simulink model "SIFT_final"  (R2015a)
settings: Solver=ode45  StartTime=0.0  StopTime=10.0  RelTol=1e-3
InitFcn:
  | %% DSPBuilder Start
  | alt_dspbuilder_update_model(bdroot)
  | %% DSPBuilder End
libraries: allblocks_alteradspbuilder2 x1826
(part 1 of 24)
settings Model: Creator=ASUS  LastModifiedBy=ASUS

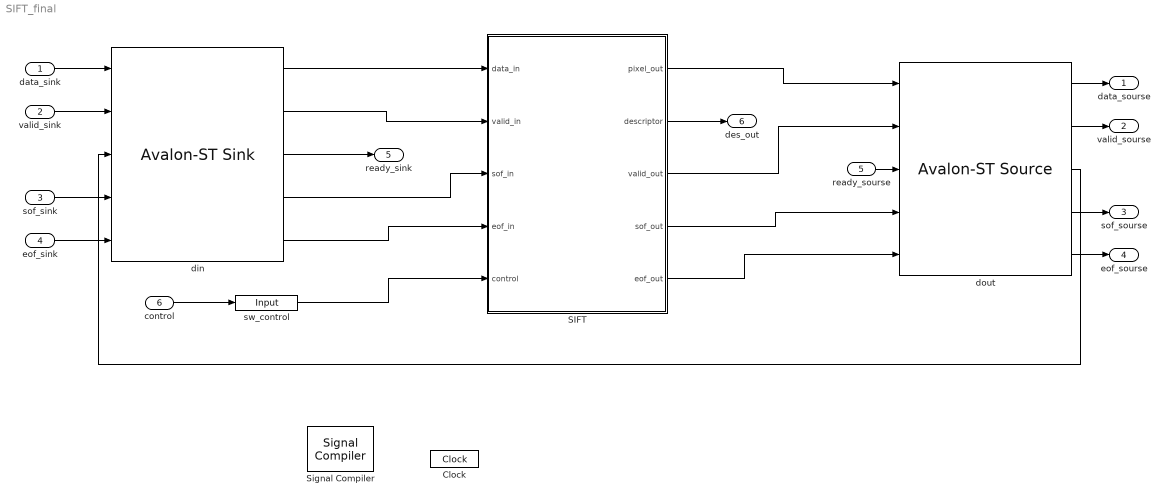
== system SIFT_final ==
  data_sink : Inport
  valid_sink : Inport  Port=2
  sof_sink : Inport  Port=3
  eof_sink : Inport  Port=4
  ready_sourse : Inport  Port=5
  control : Inport  Port=6
  Clock : allblocks_alteradspbuilder2/Clock  ClockPeriod=10/1.5  ClockPeriodUnit=ns  SampleTime=1  ResetLatency=0  ResetRegisterCascadeDepth=0  SimulationStartCycle=5  PhaseOffset=0  Reset=aclr  ResetType=Active Low  Export=off
  SIFT : Subsystem
  Signal Compiler : allblocks_alteradspbuilder2/Signal Compiler  DeviceFamily=Cyclone IV GX  DeviceName=AUTO  DisableEarlyHDLGeneration=off  EnableSignalTap=on  SignalTapDepth=256  UseBoardBlock=off  StpUseDefaultClock=on  StpClock=Clock  ExportDir=C:\altera\16.0\quartus\dsp_builder  MAX10_ProgrammingMode=Internal Flash (SDM) Single Boot
  din : allblocks_alteradspbuilder2/Avalon-ST Sink  iofile=C:\Users\ASUS\Desktop\final_sift_fpga\tb_SIFT_final\SIFT%5Ffinal_din_data.salt,C:\Users\ASUS\Desktop\final_sift_fpga\tb_SIFT_final\SIFT%5Ffinal_din_valid.salt,C:\Users\ASUS\Desktop\final_sift_fpga\tb_SIFT_final\SIFT%5Ffinal_din_ready.capture,C:\Users\ASUS\Desktop\final_sift_fpga\tb_SIFT_final\SIFT%5Ffinal_din_startofpacket.salt,C:\Users\ASUS\Desktop\final_sift_fpga\tb_SIFT_final\SIFT%5Ffinal_din_endofpacket.salt,  SpecifyClock=off  BusType=Unsigned Integer  bwl=24  bwr=0  symbolWidth=8  symbolsPerBeat=3  numOfChannels=0  numOfErrorDescriptors=0  endOfPacket=on  startOfPacket=on  empty=off  readyLatency=1  externalType=Inferred  PORTTYPE=Output
  dout : allblocks_alteradspbuilder2/Avalon-ST Source  iofile=C:\Users\ASUS\Desktop\final_sift_fpga\tb_SIFT_final\SIFT%5Ffinal_dout_data.capture,C:\Users\ASUS\Desktop\final_sift_fpga\tb_SIFT_final\SIFT%5Ffinal_dout_valid.capture,C:\Users\ASUS\Desktop\final_sift_fpga\tb_SIFT_final\SIFT%5Ffinal_dout_ready.salt,C:\Users\ASUS\Desktop\final_sift_fpga\tb_SIFT_final\SIFT%5Ffinal_dout_startofpacket.capture,C:\Users\ASUS\Desktop\final_sift_fpga\tb_SIFT_final\SIFT%5Ffinal_dout_endofpacket.capture,  SpecifyClock=off  BusType=Unsigned Integer  bwl=24  bwr=0  symbolWidth=8  symbolsPerBeat=3  numOfChannels=0  numOfErrorDescriptors=0  endOfPacket=on  startOfPacket=on  empty=off  readyLatency=1  externalType=Inferred  PORTTYPE=Input
  sw_control : allblocks_alteradspbuilder2/Input  iofile=C:\Users\ASUS\Desktop\final_sift_fpga\tb_SIFT_final\SIFT%5Ffinal_sw%5Fcontrol.salt  BusType=Unsigned Integer  bwl=18  bwr=0  SpecifyClock=off  PORTTYPE=Input  externalType=Inferred  allowFloatingPointOverride=on  logOutputs=off
  data_sourse : Outport
  valid_sourse : Outport  Port=2
  sof_sourse : Outport  Port=3
  eof_sourse : Outport  Port=4
  ready_sink : Outport  Port=5
  des_out : Outport  Port=6
  wires:
  SIFT/1(pixel_out) -> dout/1
  din/1 -> SIFT/1(data_in)
  din/2 -> SIFT/2(valid_in)
  SIFT/3(valid_out) -> dout/2
  SIFT/4(sof_out) -> dout/4
  SIFT/5(eof_out) -> dout/5
  din/5 -> SIFT/4(eof_in)
  din/4 -> SIFT/3(sof_in)
  dout/3 -> din/3
  dout/1 -> data_sourse/1
  dout/2 -> valid_sourse/1
  dout/4 -> sof_sourse/1
  dout/5 -> eof_sourse/1
  data_sink/1 -> din/1
  valid_sink/1 -> din/2
  sof_sink/1 -> din/4
  eof_sink/1 -> din/5
  ready_sourse/1 -> dout/3
  din/3 -> ready_sink/1
  control/1 -> sw_control/1
  sw_control/1 -> SIFT/5(control)
  SIFT/2(descriptor) -> des_out/1

== system SIFT_final/SIFT ==
  data_in : Inport
  valid_in : Inport  Port=2
  sof_in : Inport  Port=3
  eof_in : Inport  Port=4
  control : Inport  Port=5
  Calculate_descriptor : Subsystem
  Memory Delay : allblocks_alteradspbuilder2/Memory Delay  BusType=Inferred  bwl=8  bwr=0  pipeline=2581  pipeline_display=2581  ram_type=AUTO  use_ena=on  use_sclr=off  allowFloatingPointOverride=on  logOutputs=off  logFile=C:\Users\ASUS\Desktop\final_sift_fpga\tb_SIFT_final\SIFT%5Ffinal_SIFT_Memory+Delay.fixedpointlog
  Memory Delay1 : allblocks_alteradspbuilder2/Memory Delay  BusType=Inferred  bwl=8  bwr=0  pipeline=2581  pipeline_display=2581  ram_type=AUTO  use_ena=on  use_sclr=off  allowFloatingPointOverride=on  logOutputs=off  logFile=C:\Users\ASUS\Desktop\final_sift_fpga\tb_SIFT_final\SIFT%5Ffinal_SIFT_Memory+Delay1.fixedpointlog
  Memory Delay2 : allblocks_alteradspbuilder2/Memory Delay  BusType=Inferred  bwl=8  bwr=0  pipeline=6477+26  pipeline_display=6503  ram_type=AUTO  use_ena=on  use_sclr=off  allowFloatingPointOverride=on  logOutputs=off  logFile=C:\Users\ASUS\Desktop\final_sift_fpga\tb_SIFT_final\SIFT%5Ffinal_SIFT_Memory+Delay2.fixedpointlog
  Memory Delay3 : allblocks_alteradspbuilder2/Memory Delay  BusType=Inferred  bwl=8  bwr=0  pipeline=2581+5180  pipeline_display=7761  ram_type=AUTO  use_ena=on  use_sclr=off  allowFloatingPointOverride=on  logOutputs=off  logFile=C:\Users\ASUS\Desktop\final_sift_fpga\tb_SIFT_final\SIFT%5Ffinal_SIFT_Memory+Delay3.fixedpointlog
  Memory Delay4 : allblocks_alteradspbuilder2/Memory Delay  BusType=Inferred  bwl=8  bwr=0  pipeline=2581+5180  pipeline_display=7761  ram_type=AUTO  use_ena=on  use_sclr=off  allowFloatingPointOverride=on  logOutputs=off  logFile=C:\Users\ASUS\Desktop\final_sift_fpga\tb_SIFT_final\SIFT%5Ffinal_SIFT_Memory+Delay4.fixedpointlog
  Memory Delay5 : allblocks_alteradspbuilder2/Memory Delay  BusType=Inferred  bwl=8  bwr=0  pipeline=26  pipeline_display=26  ram_type=AUTO  use_ena=on  use_sclr=off  allowFloatingPointOverride=on  logOutputs=off  logFile=C:\Users\ASUS\Desktop\final_sift_fpga\tb_SIFT_final\SIFT%5Ffinal_SIFT_Memory+Delay5.fixedpointlog
  Memory Delay6 : allblocks_alteradspbuilder2/Memory Delay  BusType=Inferred  bwl=8  bwr=0  pipeline=26  pipeline_display=26  ram_type=AUTO  use_ena=on  use_sclr=off  allowFloatingPointOverride=on  logOutputs=off  logFile=C:\Users\ASUS\Desktop\final_sift_fpga\tb_SIFT_final\SIFT%5Ffinal_SIFT_Memory+Delay6.fixedpointlog
  RGB2GRAY : Subsystem
  SIFT_detector : Subsystem
  Show_keypoint : Subsystem
  pixel_out : Outport
  descriptor : Outport  Port=2
  valid_out : Outport  Port=3
  sof_out : Outport  Port=4
  eof_out : Outport  Port=5
  wires:
  Memory Delay4/1 -> eof_out/1
  Memory Delay3/1 -> sof_out/1
  [eof_in] -> Memory Delay4/1
  [sof_in] -> Memory Delay3/1
  [valid_in] -> Memory Delay3/2
  [valid_in] -> valid_out/1
  [valid_in] -> Memory Delay4/2
  valid_in/1 -> Memory Delay5/2, Memory Delay6/2, RGB2GRAY/2(clken), [valid_in]
  control/1 -> [control]
  RGB2GRAY/1(gray) -> SIFT_detector/1(data_in)
  [valid_in] -> Calculate_descriptor/2(valid_in), SIFT_detector/2(valid_in)
  [sof_in] -> SIFT_detector/3(sof_in)
  [eof_in] -> Calculate_descriptor/3(eof_in), SIFT_detector/4(eof_in)
  SIFT_detector/3(scale2) -> Calculate_descriptor/1(data_in)
  SIFT_detector/1(iskeypoint1) -> Memory Delay/1
  Calculate_descriptor/1(descriptor_out) -> descriptor/1
  Memory Delay/1 -> Show_keypoint/1(iskeypoint_oct1)
  SIFT_detector/2(iskeypoint0) -> Memory Delay1/1
  Memory Delay1/1 -> Show_keypoint/2(iskeypoint_oct0)
  Show_keypoint/1(pixel_out) -> pixel_out/1
  [valid_in] -> Memory Delay2/2, Memory Delay1/2, Memory Delay/2, Show_keypoint/3(valid_in)
  [control] -> Show_keypoint/4(control)
  data_in/1 -> Memory Delay2/1, RGB2GRAY/1("pixel_in ")
  Memory Delay2/1 -> Show_keypoint/5(data_in)
  eof_in/1 -> Memory Delay6/1
  sof_in/1 -> Memory Delay5/1
  Memory Delay5/1 -> [sof_in]
  Memory Delay6/1 -> [eof_in]

== system SIFT_final/SIFT/Calculate_descriptor ==
  data_in : Inport
  valid_in : Inport  Port=2
  eof_in : Inport  Port=3
  AltBus5 : allblocks_alteradspbuilder2/AltBus  BusType=Unsigned Integer  bwl=8  bwr=0  saturate=off  floatingPointInput=on  floatingPointOutput=on  logOutputs=off  logFile=C:\Users\ASUS\Desktop\final_sift_fpga\tb_SIFT_final\SIFT%5Ffinal_SIFT_Calculate%5Fdescriptor_AltBus5.fixedpointlog
  AltBus6 : allblocks_alteradspbuilder2/AltBus  BusType=Unsigned Fractional  bwl=10  bwr=16  saturate=off  floatingPointInput=on  floatingPointOutput=on  logOutputs=off  logFile=C:\Users\ASUS\Desktop\final_sift_fpga\tb_SIFT_final\SIFT%5Ffinal_SIFT_Calculate%5Fdescriptor_AltBus6.fixedpointlog
  GradOrien : Subsystem
  Line_buff_11x11 : Subsystem
  Memory Delay1 : allblocks_alteradspbuilder2/Memory Delay  BusType=Inferred  bwl=8  bwr=0  pipeline=3206  pipeline_display=3206  ram_type=AUTO  use_ena=on  use_sclr=off  allowFloatingPointOverride=on  logOutputs=off  logFile=C:\Users\ASUS\Desktop\final_sift_fpga\tb_SIFT_final\SIFT%5Ffinal_SIFT_Calculate%5Fdescriptor_Memory+Delay1.fixedpointlog
  Memory Delay2 : allblocks_alteradspbuilder2/Memory Delay  BusType=Inferred  bwl=8  bwr=0  pipeline=6477  pipeline_display=6477  ram_type=AUTO  use_ena=on  use_sclr=off  allowFloatingPointOverride=on  logOutputs=off  logFile=C:\Users\ASUS\Desktop\final_sift_fpga\tb_SIFT_final\SIFT%5Ffinal_SIFT_Calculate%5Fdescriptor_Memory+Delay2.fixedpointlog
  Round : allblocks_alteradspbuilder2/Round  BusType=Unsigned Fractional  bwl=8  bwr=16  bitsToRemove=0  roundMode=TRUNCATE_LOW  userRoundMode=Truncate  pipeline=off  pipeline_display=0  use_ena=off  use_aclr=off
  descriptor : Subsystem
  hist_bin : Subsystem
  descriptor_out : Outport
  wires:
  AltBus5/1 -> hist_bin/2(orien_In)
  GradOrien/1(m_xy) -> AltBus6/1
  GradOrien/2(orien) -> AltBus5/1
  valid_in/1 -> GradOrien/2(clken), Memory Delay2/2, Memory Delay1/2, Line_buff_11x11/2(clken), descriptor/10(valid_in), hist_bin/3(clken)
  Round/1 -> GradOrien/1(data_in)
  AltBus6/1 -> hist_bin/1(m_xy_In)
  data_in/1 -> Round/1
  Line_buff_11x11/1(Out00) -> descriptor/1(data_in00)
  Line_buff_11x11/2(Out05) -> descriptor/2(data_in05)
  Line_buff_11x11/3(Out010) -> descriptor/3(data_in010)
  Line_buff_11x11/4(Out50) -> descriptor/4(data_in50)
  Line_buff_11x11/5(Out55) -> descriptor/5(data_in55)
  Line_buff_11x11/6(Out510) -> descriptor/6(data_in510)
  Line_buff_11x11/7(Out100) -> descriptor/7(data_in100)
  Line_buff_11x11/8(Out105) -> descriptor/8(data_in105)
  Line_buff_11x11/9(Out1010) -> descriptor/9(data_in1010)
  hist_bin/1(hist_bin_out) -> Line_buff_11x11/1(dataIn)
  hist_bin/2(Orien_out) -> Memory Delay1/1
  Memory Delay1/1 -> descriptor/11(orien_in)
  descriptor/1(descriptor_out) -> descriptor_out/1
  eof_in/1 -> Memory Delay2/1
  Memory Delay2/1 -> descriptor/12(eof_in)

== system SIFT_final/SIFT/RGB2GRAY ==
  "pixel_in " : Inport
  clken : Inport  Port=2
  AltBus : allblocks_alteradspbuilder2/AltBus  BusType=Unsigned Integer  bwl=8  bwr=0  saturate=off  floatingPointInput=on  floatingPointOutput=on  logOutputs=off  logFile=C:\Users\ASUS\Desktop\final_sift_fpga\tb_SIFT_final\SIFT%5Ffinal_SIFT_RGB2GRAY_AltBus.fixedpointlog
  Bus Conversion : allblocks_alteradspbuilder2/Bus Conversion  BusType=Unsigned Integer  ibwl=24  ibwr=1  bwl=8  bwr=1  bitToConnectToOutputLSB=16  round=off  saturate=off  pipeline_display=0
  Bus Conversion1 : allblocks_alteradspbuilder2/Bus Conversion  BusType=Unsigned Integer  ibwl=24  ibwr=1  bwl=8  bwr=1  bitToConnectToOutputLSB=8  round=off  saturate=off  pipeline_display=0
  Bus Conversion2 : allblocks_alteradspbuilder2/Bus Conversion  BusType=Unsigned Integer  ibwl=24  ibwr=1  bwl=8  bwr=1  bitToConnectToOutputLSB=0  round=off  saturate=off  pipeline_display=0
  Constant : allblocks_alteradspbuilder2/Constant  mask_cst=16  BusType=Unsigned Integer  bwl=8  bwr=0  roundMode=Truncate  satMode=Wrap  SpecifyClock=off  allowFloatingPointOverride=on  logOutputs=off  logFile=C:\Users\ASUS\Desktop\final_sift_fpga\tb_SIFT_final\SIFT%5Ffinal_SIFT_RGB2GRAY_Constant.fixedpointlog
  Gain : allblocks_alteradspbuilder2/Gain  vgain=0.257  BusType=Unsigned Fractional  bwl=8  bwr=16  pipeline=24  pipeline_display=24  allowFloatingPointOverride=on  logOutputs=off  logFile=C:\Users\ASUS\Desktop\final_sift_fpga\tb_SIFT_final\SIFT%5Ffinal_SIFT_RGB2GRAY_Gain.fixedpointlog  use_ena=on  use_aclr=off  lpm=off  MaskValue=1
  Gain1 : allblocks_alteradspbuilder2/Gain  vgain=0.504  BusType=Unsigned Fractional  bwl=8  bwr=16  pipeline=24  pipeline_display=24  allowFloatingPointOverride=on  logOutputs=off  logFile=C:\Users\ASUS\Desktop\final_sift_fpga\tb_SIFT_final\SIFT%5Ffinal_SIFT_RGB2GRAY_Gain1.fixedpointlog  use_ena=on  use_aclr=off  lpm=off  MaskValue=1
  Gain2 : allblocks_alteradspbuilder2/Gain  vgain=0.098  BusType=Unsigned Fractional  bwl=8  bwr=16  pipeline=24  pipeline_display=24  allowFloatingPointOverride=on  logOutputs=off  logFile=C:\Users\ASUS\Desktop\final_sift_fpga\tb_SIFT_final\SIFT%5Ffinal_SIFT_RGB2GRAY_Gain2.fixedpointlog  use_ena=on  use_aclr=off  lpm=off  MaskValue=1
  Parallel Adder Subtractor : allblocks_alteradspbuilder2/Parallel Adder Subtractor  number_of_inputs=4  direction=+  use_pipeline=on  pipeline_display=2  phase_selection=1  use_ena=on  use_aclr=off  allowFloatingPointOverride=on  logOutputs=off  logFile=C:\Users\ASUS\Desktop\final_sift_fpga\tb_SIFT_final\SIFT%5Ffinal_SIFT_RGB2GRAY_Parallel+Adder+Subtractor.fixedpointlog
  gray : Outport
  wires:
  "pixel_in "/1 -> [pixel_in]
  Gain1/1 -> [G_Y]
  [clken] -> Gain1/2
  Gain2/1 -> [B_Y]
  [G_chanel] -> Gain1/1
  clken/1 -> [clken]
  [B_chanel] -> Gain2/1
  [R_chanel] -> Gain/1
  Gain/1 -> [R_Y]
  [clken] -> Gain2/2
  [clken] -> Gain/2
  [R_Y] -> Parallel Adder Subtractor/1
  [G_Y] -> Parallel Adder Subtractor/2
  [B_Y] -> Parallel Adder Subtractor/3
  [clken] -> Parallel Adder Subtractor/5
  Parallel Adder Subtractor/1 -> AltBus/1
  Constant/1 -> Parallel Adder Subtractor/4
  Bus Conversion/1 -> [R_chanel]
  Bus Conversion1/1 -> [G_chanel]
  [pixel_in] -> Bus Conversion1/1, Bus Conversion2/1, Bus Conversion/1
  Bus Conversion2/1 -> [B_chanel]
  AltBus/1 -> gray/1

== system SIFT_final/SIFT/SIFT_detector ==
  data_in : Inport
  valid_in : Inport  Port=2
  sof_in : Inport  Port=3
  eof_in : Inport  Port=4
  AltBus4 : allblocks_alteradspbuilder2/AltBus  BusType=Unsigned Integer  bwl=8  bwr=0  saturate=off  floatingPointInput=on  floatingPointOutput=on  logOutputs=off  logFile=C:\Users\ASUS\Desktop\final_sift_fpga\tb_SIFT_final\SIFT%5Ffinal_SIFT_SIFT%5Fdetector_AltBus4.fixedpointlog
  AltBus5 : allblocks_alteradspbuilder2/AltBus  BusType=Single Bit  bwl=8  bwr=0  saturate=off  floatingPointInput=on  floatingPointOutput=on  logOutputs=off  logFile=C:\Users\ASUS\Desktop\final_sift_fpga\tb_SIFT_final\SIFT%5Ffinal_SIFT_SIFT%5Fdetector_AltBus5.fixedpointlog
  AltBus6 : allblocks_alteradspbuilder2/AltBus  BusType=Single Bit  bwl=8  bwr=0  saturate=off  floatingPointInput=on  floatingPointOutput=on  logOutputs=off  logFile=C:\Users\ASUS\Desktop\final_sift_fpga\tb_SIFT_final\SIFT%5Ffinal_SIFT_SIFT%5Fdetector_AltBus6.fixedpointlog
  AltBus7 : allblocks_alteradspbuilder2/AltBus  BusType=Unsigned Integer  bwl=8  bwr=0  saturate=off  floatingPointInput=on  floatingPointOutput=on  logOutputs=off  logFile=C:\Users\ASUS\Desktop\final_sift_fpga\tb_SIFT_final\SIFT%5Ffinal_SIFT_SIFT%5Fdetector_AltBus7.fixedpointlog
  Delay3 : allblocks_alteradspbuilder2/Delay  pipeline=1948  pipeline_display=1948  ClockPhase=1  use_ena=on  use_sclr=off  allowFloatingPointOverride=on  logOutputs=off  logFile=C:\SIFT%5Ffinal_SIFT_SIFT%5Fdetector_Delay3.fixedpointlog  use_init=off  reset_value=0
  Octave0 : Subsystem
  Octave1 : Subsystem
  resize : Subsystem
  iskeypoint1 : Outport
  iskeypoint0 : Outport  Port=2
  scale2 : Outport  Port=3
  wires:
  Octave0/2(scale2) -> scale2/1
  sof_in/1 -> resize/3(sof_in)
  AltBus5/1 -> Delay3/1
  AltBus4/1 -> Octave0/1(data_in)
  Octave0/1(Out1) -> AltBus5/1
  data_in/1 -> AltBus4/1, AltBus7/1
  eof_in/1 -> resize/2(eof_in)
  Octave1/1(Out1) -> AltBus6/1
  resize/1(select) -> Octave1/2(valid_in)
  valid_in/1 -> Delay3/2, Octave0/2(valid_in), resize/1(valid_in)
  AltBus7/1 -> Octave1/1(data_in)
  AltBus6/1 -> iskeypoint1/1
  Delay3/1 -> iskeypoint0/1

== system SIFT_final/SIFT/Show_keypoint ==
  iskeypoint_oct1 : Inport
  iskeypoint_oct0 : Inport  Port=2
  valid_in : Inport  Port=3
  control : Inport  Port=4
  data_in : Inport  Port=5
  AltBus : allblocks_alteradspbuilder2/AltBus  BusType=Unsigned Integer  bwl=2  bwr=0  saturate=off  floatingPointInput=on  floatingPointOutput=on  logOutputs=off  logFile=C:\Users\ASUS\Desktop\final_sift_fpga\tb_SIFT_final\SIFT%5Ffinal_SIFT_Show%5Fkeypoint_AltBus.fixedpointlog
  Delay1 : allblocks_alteradspbuilder2/Delay  pipeline=642  pipeline_display=642  ClockPhase=1  use_ena=on  use_sclr=off  allowFloatingPointOverride=on  logOutputs=off  logFile=C:\Users\ASUS\Desktop\final_sift_fpga\tb_SIFT_final\SIFT%5Ffinal_SIFT_Show%5Fkeypoint_Delay1.fixedpointlog  use_init=off  reset_value=1
  Delay2 : allblocks_alteradspbuilder2/Delay  pipeline=1  pipeline_display=1  ClockPhase=1  use_ena=on  use_sclr=off  allowFloatingPointOverride=on  logOutputs=off  logFile=C:\Users\ASUS\Desktop\final_sift_fpga\tb_SIFT_final\SIFT%5Ffinal_SIFT_Show%5Fkeypoint_Delay2.fixedpointlog  use_init=off  reset_value=1
  Logical Bit Operator1 : allblocks_alteradspbuilder2/Logical Bit Operator  LogicalOperator=OR  user_inputs=2  pipeline_display=0
  Multiplexer1 : allblocks_alteradspbuilder2/Multiplexer  numInputs=3  pipeline=1  oneHot=off  pipeline_display=1  use_ena=on  use_aclr=off  allowFloatingPointOverride=on  logOutputs=off  logFile=C:\Users\ASUS\Desktop\final_sift_fpga\tb_SIFT_final\SIFT%5Ffinal_SIFT_Show%5Fkeypoint_Multiplexer1.fixedpointlog
  show_key : Subsystem
  pixel_out : Outport
  wires:
  iskeypoint_oct0/1 -> [octave1]
  Logical Bit Operator1/1 -> Multiplexer1/2
  valid_in/1 -> [valid_in]
  control/1 -> [control]
  iskeypoint_oct1/1 -> [octave2]
  data_in/1 -> [data_in]
  [octave1] -> Multiplexer1/3, Logical Bit Operator1/1
  [octave2] -> Multiplexer1/4, Logical Bit Operator1/2
  AltBus/1 -> Multiplexer1/1
  [control] -> AltBus/1
  [valid_in] -> Delay2/2, Delay1/2, show_key/3(clken), Multiplexer1/5
  show_key/1(Out) -> pixel_out/1
  Multiplexer1/1 -> Delay1/1
  [data_in] -> Delay2/1
  Delay2/1 -> show_key/1(dataIn)
  Delay1/1 -> show_key/2("is_keypoint ")

== system SIFT_final/SIFT/Calculate_descriptor/GradOrien ==
  data_in : Inport
  clken : Inport  Port=2
  lineBuff_3x3 : Subsystem
  sub_GradOrian : Subsystem
  m_xy : Outport
  orien : Outport  Port=2
  wires:
  sub_GradOrian/1(orien) -> orien/1
  clken/1 -> sub_GradOrian/5(clken), lineBuff_3x3/2(clken)
  data_in/1 -> lineBuff_3x3/1(dataIn)
  sub_GradOrian/2(m_xy) -> m_xy/1
  lineBuff_3x3/1(Out01) -> sub_GradOrian/1(L_y_add_1)
  lineBuff_3x3/4(Out21) -> sub_GradOrian/4(L_y_sub_1)
  lineBuff_3x3/3(Out12) -> sub_GradOrian/3(L_x_sub_1)
  lineBuff_3x3/2(Out10) -> sub_GradOrian/2(L_x_add_1)

== system SIFT_final/SIFT/Calculate_descriptor/Line_buff_11x11 ==
  dataIn : Inport
  clken : Inport  Port=2
  Memory Delay1 : allblocks_alteradspbuilder2/Memory Delay  BusType=Unsigned Integer  bwl=128  bwr=0  pipeline=1  pipeline_display=1  ram_type=AUTO  use_ena=on  use_sclr=off  allowFloatingPointOverride=on  logOutputs=off  logFile=C:\Users\ASUS\Desktop\final_sift_fpga\tb_SIFT_final\SIFT%5Ffinal_SIFT_Calculate%5Fdescriptor_Line%5Fbuff%5F11x11_Memory+Delay1.fixedpointlog
  Memory Delay11 : allblocks_alteradspbuilder2/Memory Delay  BusType=Inferred  bwl=128  bwr=0  pipeline=630  pipeline_display=630  ram_type=AUTO  use_ena=on  use_sclr=off  allowFloatingPointOverride=on  logOutputs=off  logFile=C:\Users\ASUS\Desktop\final_sift_fpga\tb_SIFT_final\SIFT%5Ffinal_SIFT_Calculate%5Fdescriptor_Line%5Fbuff%5F11x11_Memory+Delay11.fixedpointlog
  Memory Delay12 : allblocks_alteradspbuilder2/Memory Delay  BusType=Inferred  bwl=128  bwr=0  pipeline=5  pipeline_display=5  ram_type=AUTO  use_ena=on  use_sclr=off  allowFloatingPointOverride=on  logOutputs=off  logFile=C:\Users\ASUS\Desktop\final_sift_fpga\tb_SIFT_final\SIFT%5Ffinal_SIFT_Calculate%5Fdescriptor_Line%5Fbuff%5F11x11_Memory+Delay12.fixedpointlog
  Memory Delay13 : allblocks_alteradspbuilder2/Memory Delay  BusType=Inferred  bwl=128  bwr=0  pipeline=5  pipeline_display=5  ram_type=AUTO  use_ena=on  use_sclr=off  allowFloatingPointOverride=on  logOutputs=off  logFile=C:\Users\ASUS\Desktop\final_sift_fpga\tb_SIFT_final\SIFT%5Ffinal_SIFT_Calculate%5Fdescriptor_Line%5Fbuff%5F11x11_Memory+Delay13.fixedpointlog
  Memory Delay15 : allblocks_alteradspbuilder2/Memory Delay  BusType=Inferred  bwl=128  bwr=0  pipeline=630  pipeline_display=630  ram_type=AUTO  use_ena=on  use_sclr=off  allowFloatingPointOverride=on  logOutputs=off  logFile=C:\Users\ASUS\Desktop\final_sift_fpga\tb_SIFT_final\SIFT%5Ffinal_SIFT_Calculate%5Fdescriptor_Line%5Fbuff%5F11x11_Memory+Delay15.fixedpointlog
  Memory Delay16 : allblocks_alteradspbuilder2/Memory Delay  BusType=Inferred  bwl=128  bwr=0  pipeline=5  pipeline_display=5  ram_type=AUTO  use_ena=on  use_sclr=off  allowFloatingPointOverride=on  logOutputs=off  logFile=C:\Users\ASUS\Desktop\final_sift_fpga\tb_SIFT_final\SIFT%5Ffinal_SIFT_Calculate%5Fdescriptor_Line%5Fbuff%5F11x11_Memory+Delay16.fixedpointlog
  Memory Delay17 : allblocks_alteradspbuilder2/Memory Delay  BusType=Inferred  bwl=128  bwr=0  pipeline=5  pipeline_display=5  ram_type=AUTO  use_ena=on  use_sclr=off  allowFloatingPointOverride=on  logOutputs=off  logFile=C:\Users\ASUS\Desktop\final_sift_fpga\tb_SIFT_final\SIFT%5Ffinal_SIFT_Calculate%5Fdescriptor_Line%5Fbuff%5F11x11_Memory+Delay17.fixedpointlog
  Memory Delay18 : allblocks_alteradspbuilder2/Memory Delay  BusType=Inferred  bwl=128  bwr=0  pipeline=640*4  pipeline_display=2560  ram_type=AUTO  use_ena=on  use_sclr=off  allowFloatingPointOverride=on  logOutputs=off  logFile=C:\Users\ASUS\Desktop\final_sift_fpga\tb_SIFT_final\SIFT%5Ffinal_SIFT_Calculate%5Fdescriptor_Line%5Fbuff%5F11x11_Memory+Delay18.fixedpointlog
  Memory Delay5 : allblocks_alteradspbuilder2/Memory Delay  BusType=Inferred  bwl=128  bwr=0  pipeline=5  pipeline_display=5  ram_type=AUTO  use_ena=on  use_sclr=off  allowFloatingPointOverride=on  logOutputs=off  logFile=C:\Users\ASUS\Desktop\final_sift_fpga\tb_SIFT_final\SIFT%5Ffinal_SIFT_Calculate%5Fdescriptor_Line%5Fbuff%5F11x11_Memory+Delay5.fixedpointlog
  Memory Delay6 : allblocks_alteradspbuilder2/Memory Delay  BusType=Inferred  bwl=128  bwr=0  pipeline=5  pipeline_display=5  ram_type=AUTO  use_ena=on  use_sclr=off  allowFloatingPointOverride=on  logOutputs=off  logFile=C:\Users\ASUS\Desktop\final_sift_fpga\tb_SIFT_final\SIFT%5Ffinal_SIFT_Calculate%5Fdescriptor_Line%5Fbuff%5F11x11_Memory+Delay6.fixedpointlog
  Memory Delay7 : allblocks_alteradspbuilder2/Memory Delay  BusType=Inferred  bwl=128  bwr=0  pipeline=640*4  pipeline_display=2560  ram_type=AUTO  use_ena=on  use_sclr=off  allowFloatingPointOverride=on  logOutputs=off  logFile=C:\Users\ASUS\Desktop\final_sift_fpga\tb_SIFT_final\SIFT%5Ffinal_SIFT_Calculate%5Fdescriptor_Line%5Fbuff%5F11x11_Memory+Delay7.fixedpointlog
  Out00 : Outport
  Out05 : Outport  Port=2
  Out010 : Outport  Port=3
  Out50 : Outport  Port=4
  Out55 : Outport  Port=5
  Out510 : Outport  Port=6
  Out100 : Outport  Port=7
  Out105 : Outport  Port=8
  Out1010 : Outport  Port=9
  wires:
  [clken] -> Memory Delay11/2
  [clken] -> Memory Delay17/2
  [clken] -> Memory Delay6/2
  Memory Delay6/1 -> [data_010], Memory Delay7/1
  [clken] -> Memory Delay18/2
  Memory Delay18/1 -> Memory Delay15/1
  Memory Delay13/1 -> Memory Delay18/1, [data_510]
  [clken] -> Memory Delay15/2
  [clken] -> Memory Delay16/2
  Memory Delay17/1 -> [data_1010]
  Memory Delay16/1 -> Memory Delay17/1, [data_105]
  Memory Delay15/1 -> Memory Delay16/1, [data_100]
  [clken] -> Memory Delay7/2
  [clken] -> Memory Delay12/2
  Memory Delay11/1 -> Memory Delay12/1, [data_50]
  Memory Delay12/1 -> Memory Delay13/1, [data_55]
  Memory Delay7/1 -> Memory Delay11/1
  [clken] -> Memory Delay13/2
  [data_55] -> Out55/1
  [data_010] -> Out010/1
  [data_05] -> Out05/1
  clken/1 -> [clken]
  [data_00] -> Out00/1
  [data_50] -> Out50/1
  [data_100] -> Out100/1
  [data_510] -> Out510/1
  [data_1010] -> Out1010/1
  dataIn/1 -> [data_in]
  [data_105] -> Out105/1
  [clken] -> Memory Delay5/2
  Memory Delay1/1 -> Memory Delay5/1, [data_00]
  [clken] -> Memory Delay1/2
  [data_in] -> Memory Delay1/1
  Memory Delay5/1 -> Memory Delay6/1, [data_05]

== system SIFT_final/SIFT/Calculate_descriptor/descriptor ==
  data_in00 : Inport
  data_in05 : Inport  Port=2
  data_in010 : Inport  Port=3
  data_in50 : Inport  Port=4
  data_in55 : Inport  Port=5
  data_in510 : Inport  Port=6
  data_in100 : Inport  Port=7
  data_in105 : Inport  Port=8
  data_in1010 : Inport  Port=9
  valid_in : Inport  Port=10
  orien_in : Inport  Port=11
  eof_in : Inport  Port=12
  Bus Concatenation : allblocks_alteradspbuilder2/Bus Concatenation  isSigned=off  awidth=10  bwidth=10  pipeline_display=0
  Bus Concatenation1 : allblocks_alteradspbuilder2/Bus Concatenation  isSigned=off  awidth=20  bwidth=1152  pipeline_display=0
  Multiplexer : allblocks_alteradspbuilder2/Multiplexer  numInputs=8  pipeline=0  oneHot=off  pipeline_display=0  use_ena=off  use_aclr=off  allowFloatingPointOverride=on  logOutputs=off  logFile=C:\Users\ASUS\Desktop\final_sift_fpga\tb_SIFT_final\SIFT%5Ffinal_SIFT_Calculate%5Fdescriptor_descriptor_Multiplexer.fixedpointlog
  counter : Subsystem
  descriptor : Subsystem
  descriptor_out : Outport
  wires:
  valid_in/1 -> [valid_in]
  data_in1010/1 -> [hist_1010]
  data_in105/1 -> [hist_105]
  data_in100/1 -> [hist_100]
  data_in510/1 -> [hist_510]
  data_in50/1 -> [hist_50]
  data_in010/1 -> [hist_010]
  data_in05/1 -> [hist_05]
  data_in00/1 -> [hist_00]
  data_in55/1 -> [hist_55]
  orien_in/1 -> [select]
  [hist_105] -> descriptor/8(data_in8)
  [hist_100] -> descriptor/7(data_in7)
  [hist_510] -> descriptor/6(data_in6)
  [hist_55] -> descriptor/5(data_in5)
  [hist_1010] -> descriptor/9(data_in9)
  [hist_05] -> descriptor/2(data_in2)
  [hist_010] -> descriptor/3(data_in3)
  [hist_50] -> descriptor/4(data_in4)
  [hist_00] -> descriptor/1(data_in1)
  descriptor/1(descriptor1) -> Multiplexer/2
  descriptor/2(descriptor2) -> Multiplexer/3
  descriptor/3(descriptor3) -> Multiplexer/4
  descriptor/4(descriptor4) -> Multiplexer/5
  descriptor/5(descriptor5) -> Multiplexer/6
  descriptor/6(descriptor6) -> Multiplexer/7
  descriptor/7(descriptor7) -> Multiplexer/8
  descriptor/8(descriptor8) -> Multiplexer/9
  [select] -> Multiplexer/1
  Multiplexer/1 -> Bus Concatenation1/2
  eof_in/1 -> [eof_in]
  [valid_in] -> counter/1(valid_in)
  [eof_in] -> counter/2(eof_in)
  counter/2(col_out) -> Bus Concatenation/2
  counter/1(row_out) -> Bus Concatenation/1
  Bus Concatenation/1 -> Bus Concatenation1/1
  Bus Concatenation1/1 -> descriptor_out/1
